simulink model "abs_error"  (R2021b)
settings: Solver=VariableStepAuto  StartTime=0.0  StopTime=10.0  RelTol=1e-3
undefined symbols (not defined in the file): magnitude, Newton, Raphson
libraries: simulink x15
settings Model: PauseTimes=1  Creator=user  LastModifiedBy=cemery

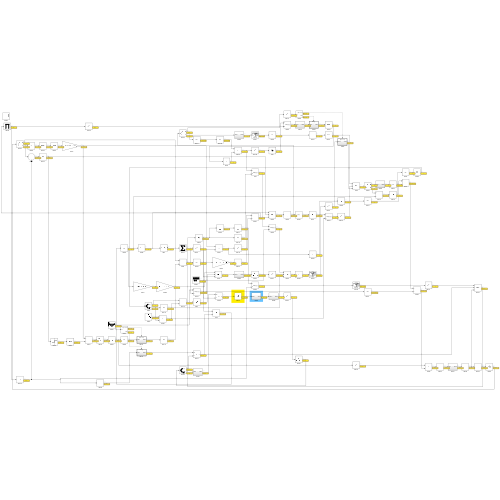
[thumbnail: Simulink's stored preview of the top-level diagram]
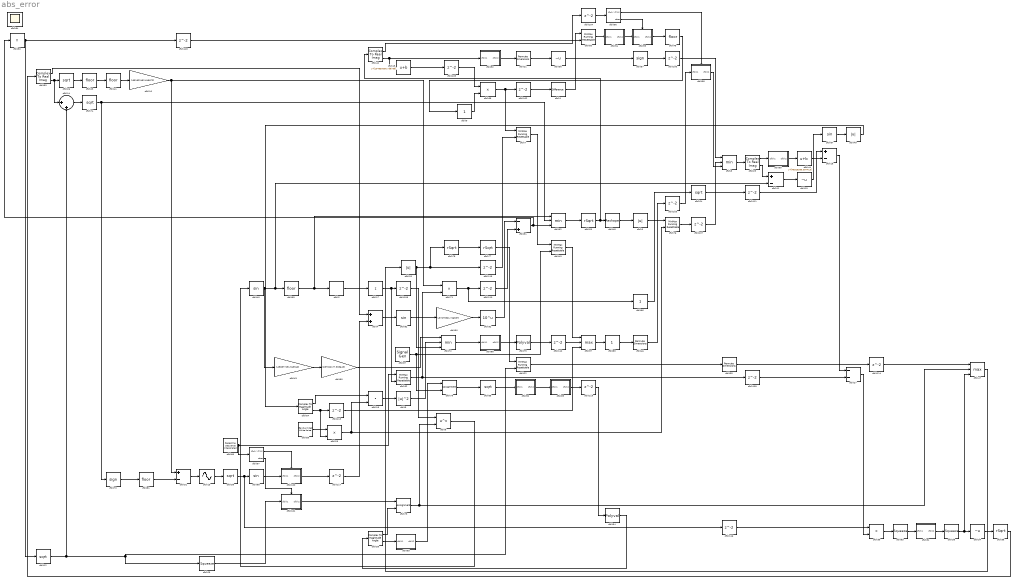
== system abs_error ==
  cfblk1 : simulink/Discrete/Difference  ICPrevInput=0.0  OutMin=[]  OutMax=[]  OutDataTypeStr=Inherit: Inherit via back propagation  OutDataType=fixdt(1, 16)  OutScaling=2^-10  DoSatur=off
  cfblk10 : Gain  Gain=[-531822452.645872]
  cfblk100 : Subsystem  TreatAsAtomicUnit=on
  cfblk101 : Subsystem  TreatAsAtomicUnit=on
  cfblk{102..119} (18 alike) : Delay  SampleTime=1
  cfblk11 : Sum  Inputs=+-
  cfblk{12,24,26,59,65,74} (6 alike) : Sqrt  SaturateOnIntegerOverflow=on
  cfblk13 : Sin  TimeSource=Use external signal  SampleTime=0
  cfblk14 : Sum  Inputs=|++
  cfblk15 : Bias  Bias=[104830006.738759]
  cfblk16 : Sum  Inputs=+-
  cfblk17 : Sum  Inputs=+
  cfblk18 : DotProduct  InputSameDT=on  OutDataTypeStr=Inherit: Inherit via internal rule
  cfblk19 : UnaryMinus
  cfblk2 : DiscreteStateSpace
  cfblk20 : Abs
  cfblk21 : PermuteDimensions
  cfblk{7,22,32,43,60,76} (6 alike) : simulink/Math Operations/MinMax Running Resettable  Function=min  vinit=0.0
  cfblk{23,41,45,69,81} (5 alike) : Rounding
  cfblk25 : Squeeze
  cfblk27 : Sum  Inputs=--
  cfblk28 : Product  Inputs=**
  cfblk29 : ComplexToRealImag
  cfblk3 : Abs
  cfblk30 : Product  Inputs=*
  cfblk31 : Sum  Inputs=-+
  cfblk{33,56,77..78} (4 alike) : Sqrt  Operator=rSqrt  AlgorithmType=Newton-Raphson  SaturateOnIntegerOverflow=on
  cfblk34 : UnaryMinus
  cfblk35 : PermuteDimensions
  cfblk36 : UnaryMinus
  cfblk37 : MinMax  Function=max  Inputs=3
  cfblk38 : Squeeze
  cfblk39 : Product
  cfblk4 : Sum
  cfblk{40,67..68,82} (4 alike) : Trigonometry
  cfblk42 : ComplexToRealImag
  cfblk44 : Bias  Bias=[46526396.097413]
  cfblk46 : PermuteDimensions
  cfblk47 : MinMax  Function=max  Inputs=3
  cfblk48 : Reshape
  cfblk49 : Abs
  cfblk5 : Math  Operator=magnitude^2  SaturateOnIntegerOverflow=on
  cfblk50 : Gain  Gain=[-97079901.726537]
  cfblk51 : Sum  Inputs=+-
  cfblk52 : Math  Operator=10^u  SaturateOnIntegerOverflow=on
  cfblk53 : ComplexToRealImag
  cfblk54 : Polyval  Coefs=[ +2.081618890e-019, -1.441693666e-014, +4.719686976e-010, -8.536869453e-006, +1.621573104e-001, -8.087801117e+001 ]
  cfblk55 : ComplexToMagnitudeAngle
  cfblk57 : Signum
  cfblk58 : Product
  cfblk6 : Math  Operator=pow  SaturateOnIntegerOverflow=on
  cfblk61 : Gain  Gain=[-258877291.943940]
  cfblk62 : MinMax  Inputs=3
  cfblk63 : Squeeze
  cfblk64 : ComplexToMagnitudeAngle
  cfblk66 : simulink/Math Operations/Slider Gain  gain=1  low=0  high=2
  cfblk70 : Signum
  cfblk71 : Product  Inputs=**
  cfblk72 : MinMax  Inputs=3
  cfblk73 : Assignment  DiagnosticForDimensions=Warning  IndexOptions=Index vector (dialog)  Indices=1  OutputSizes=1
  cfblk75 : Polyval  Coefs=[ +2.081618890e-019, -1.441693666e-014, +4.719686976e-010, -8.536869453e-006, +1.621573104e-001, -8.087801117e+001 ]
  cfblk79 : Assignment  DiagnosticForDimensions=Warning  IndexOptions=Index vector (dialog)  Indices=1  OutputSizes=1
  cfblk8 : MinMax  Inputs=3
  cfblk80 : Gain  Gain=[287322177.333645]
  cfblk83 : simulink/Math Operations/Slider Gain  gain=1  low=0  high=2
  cfblk84 : Scope
      settings: Floating=on
  cfblk85 : simulink/Sources/Band-Limited White Noise  Cov=[4231754352.057434]  Ts=0.1  seed=[6656747697.000000]
  cfblk86 : simulink/Sources/Repeating Sequence Interpolated  OutValues=[842062984.296176, 159650378.742997, -714956716.092378, -557171491.799580, 214150598.543998]  TimeValues=[0 0.1 0.5 0.6 1].'  LookUpMeth=Interpolation-Use End Values  tsamp=0.01  OutMin=[]  OutMax=[]  OutDataTypeStr=double  OutputDataTypeScalingMode=double  OutDataType=fixdt(0,8)  OutScaling=2^-10
  cfblk87 : SignalGenerator  WaveForm=square  Amplitude=[478990331.282242]  Units=rad/sec
  cfblk88 : Subsystem
  cfblk89 : Subsystem
  cfblk9 : simulink/Math Operations/Slider Gain  gain=1  low=0  high=2
  cfblk90 : Subsystem
  cfblk91 : Subsystem
  cfblk92 : Subsystem
  cfblk93 : Subsystem
  cfblk94 : Subsystem
  cfblk95 : Subsystem
  cfblk96 : If  IfExpression=u1 >= 0  SampleTime=1
  cfblk97 : If  IfExpression=u1 >= 0  SampleTime=1
  cfblk98 : Subsystem  TreatAsAtomicUnit=on
  cfblk99 : Subsystem  TreatAsAtomicUnit=on
  wires:
  cfblk24/1 -> cfblk111/1
  cfblk114/1 -> cfblk47/1
  cfblk90/1(cfblk2) -> cfblk89/1(cfblk1)
  cfblk117/1 -> cfblk4/2
  cfblk111/1 -> cfblk16/1
  cfblk89/1(cfblk2) -> cfblk119/1
  cfblk35/1 -> cfblk114/1
  cfblk119/1 -> cfblk54/1
  cfblk100/1(cfblk2) -> cfblk117/1
  cfblk115/1 -> cfblk7/2
  cfblk113/1 -> cfblk37/3
  cfblk116/1 -> cfblk39/1
  cfblk118/1 -> cfblk60/2
  cfblk112/1 -> cfblk37/2
  cfblk75/1 -> cfblk112/1
  cfblk1/1 -> cfblk60/1
  cfblk110/1 -> cfblk31/2
  cfblk45/1 -> cfblk9/1
  cfblk109/1 -> cfblk27/2
  cfblk29/2 -> cfblk11/1
  cfblk108/1 -> cfblk6/1
  cfblk107/1 -> cfblk8/2
  cfblk76/1 -> cfblk107/1
  cfblk97/1 -> cfblk100/Action
  cfblk106/1 -> cfblk8/1
  cfblk57/1 -> cfblk106/1
  cfblk105/1 -> cfblk58/1
  cfblk15/1 -> cfblk105/1
  cfblk14/1 -> cfblk74/1
  cfblk64/1 -> cfblk18/1
  cfblk104/1 -> cfblk96/1
  cfblk85/1 -> cfblk28/1
  cfblk98/1(cfblk2) -> cfblk8/3
  cfblk42/1 -> cfblk104/1
  cfblk103/1 -> cfblk98/1(cfblk1)
  cfblk46/1 -> cfblk103/1
  cfblk102/1 -> cfblk1/1
  cfblk61/1 -> cfblk80/1
  cfblk97/2 -> cfblk101/Action
  cfblk81/1 -> cfblk51/2
  cfblk96/2 -> cfblk99/Action
  cfblk19/1 -> cfblk67/1
  cfblk96/1 -> cfblk98/Action
  cfblk95/1(cfblk2) -> cfblk44/1
  cfblk3/1 -> cfblk76/1
  cfblk22/1 -> cfblk35/1
  cfblk88/1(cfblk2) -> cfblk75/1
  cfblk55/2 -> cfblk93/1(cfblk1)
  cfblk50/1 -> cfblk52/1
  cfblk77/1 -> cfblk22/1
  cfblk21/1 -> cfblk36/1
  cfblk29/1 -> cfblk95/1(cfblk1)
  cfblk48/1 -> cfblk3/1
  cfblk27/1 -> cfblk39/2
  cfblk49/1 -> cfblk64/1
  cfblk5/1 -> cfblk72/2
  cfblk7/1 -> cfblk43/1
  cfblk43/1 -> cfblk37/1
  cfblk47/1 -> cfblk20/1
  cfblk25/1 -> cfblk101/1(cfblk1)
  cfblk80/1 -> cfblk72/1
  cfblk6/1 -> cfblk40/1
  cfblk2/1 -> cfblk17/1
  cfblk54/1 -> cfblk55/1
  cfblk91/1(cfblk2) -> cfblk38/1
  cfblk26/1 -> cfblk23/1
  cfblk9/1 -> cfblk58/2
  cfblk44/1 -> cfblk16/2
  cfblk18/1 -> cfblk5/1
  cfblk82/1 -> cfblk50/1
  cfblk60/1 -> cfblk94/1(cfblk1)
  cfblk37/1 -> cfblk83/1
  cfblk53/1 -> cfblk4/1
  cfblk68/1 -> cfblk100/1(cfblk1)
  cfblk55/1 -> cfblk73/2
  cfblk66/1 -> cfblk24/1
  cfblk65/1 -> cfblk90/1(cfblk1)
  cfblk23/1 -> cfblk41/1
  cfblk13/1 -> cfblk59/1
  cfblk101/1(cfblk2) -> cfblk73/1
  cfblk83/1 -> cfblk46/1
  cfblk63/1 -> cfblk91/1(cfblk1)
  cfblk67/1 -> cfblk49/1
  cfblk78/1 -> cfblk77/1
  cfblk39/1 -> cfblk63/1
  cfblk16/1 -> cfblk27/1
  cfblk92/1(cfblk2) -> cfblk21/1
  cfblk11/1 -> cfblk19/1
  cfblk8/1 -> cfblk29/1
  cfblk4/1 -> cfblk82/1
  cfblk36/1 -> cfblk57/1
  cfblk62/1 -> cfblk33/1
  cfblk52/1 -> cfblk31/1
  cfblk56/1 -> cfblk53/1
  cfblk70/1 -> cfblk81/1
  cfblk72/1 -> cfblk88/1(cfblk1)
  cfblk79/1 -> cfblk65/1
  cfblk41/1 -> cfblk10/1
  cfblk94/1(cfblk2) -> cfblk99/1(cfblk1)
  cfblk51/1 -> cfblk13/1
  cfblk34/1 -> cfblk56/1
  cfblk99/1(cfblk2) -> cfblk45/1
  cfblk93/1(cfblk2) -> cfblk79/1
  cfblk42/2 -> cfblk15/1, cfblk92/1(cfblk1)
  cfblk10/1 -> cfblk51/1, cfblk71/1
  cfblk86/1 -> cfblk97/1, cfblk32/1
  cfblk64/2 -> cfblk28/2, cfblk113/1
  cfblk31/1 -> cfblk30/1, cfblk62/3
  cfblk20/1 -> cfblk115/1, cfblk78/1, cfblk72/3
  cfblk28/1 -> cfblk76/2, cfblk18/2
  cfblk38/1 -> cfblk34/1, cfblk47/3
  cfblk53/2 -> cfblk26/1, cfblk14/1
  cfblk58/1 -> cfblk7/1, cfblk102/1
  cfblk73/1 -> cfblk6/2, cfblk47/2
  cfblk32/1 -> cfblk71/2, cfblk109/1
  cfblk17/1 -> cfblk32/2, cfblk108/1
  cfblk69/1 -> cfblk62/1, cfblk2/1
  cfblk33/1 -> cfblk42/1, cfblk48/1
  cfblk71/1 -> cfblk66/1, cfblk110/1
  cfblk59/1 -> cfblk68/1, cfblk116/1
  cfblk87/1 -> cfblk79/2, cfblk43/2
  cfblk40/1 -> cfblk69/1, cfblk11/2, cfblk61/1
  cfblk12/1 -> cfblk25/1, cfblk22/2, cfblk14/2
  cfblk30/1 -> cfblk12/1, cfblk118/1
  cfblk74/1 -> cfblk70/1, cfblk62/2

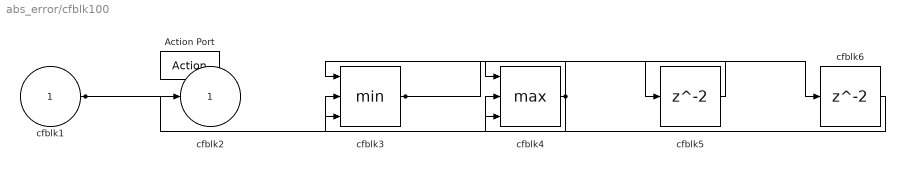
== system abs_error/cfblk100 ==
  cfblk1 : Inport
  Action Port : ActionPort  ActionPortLabel=if(u1 >= 0)
  cfblk3 : MinMax  Inputs=3
  cfblk4 : MinMax  Function=max  Inputs=3
  cfblk5 : Delay
  cfblk6 : Delay
  cfblk2 : Outport
  wires:
  cfblk1/1 -> cfblk2/1, cfblk4/2
  cfblk4/1 -> cfblk3/1, cfblk3/2, cfblk3/3
  cfblk3/1 -> cfblk5/1, cfblk6/1
  cfblk5/1 -> cfblk4/1
  cfblk6/1 -> cfblk4/3

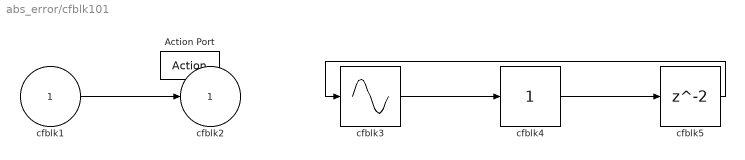
== system abs_error/cfblk101 ==
  cfblk1 : Inport
  Action Port : ActionPort  ActionPortLabel=else
  cfblk3 : Sin  TimeSource=Use external signal  SampleTime=0
  cfblk4 : simulink/Math Operations/Slider Gain  gain=1  low=0  high=2
  cfblk5 : Delay
  cfblk2 : Outport
  wires:
  cfblk3/1 -> cfblk4/1
  cfblk1/1 -> cfblk2/1
  cfblk4/1 -> cfblk5/1
  cfblk5/1 -> cfblk3/1

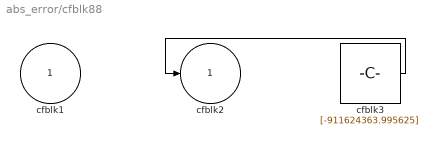
== system abs_error/cfblk88 ==
  cfblk1 : Inport
  cfblk3 : Constant  Value=[-911624363.995625]  SampleTime=1
  cfblk2 : Outport
  wires:
  cfblk3/1 -> cfblk2/1

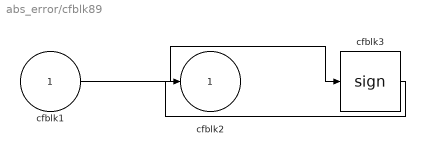
== system abs_error/cfblk89 ==
  cfblk1 : Inport
  cfblk3 : Signum
  cfblk2 : Outport
  wires:
  cfblk1/1 -> cfblk3/1
  cfblk3/1 -> cfblk2/1

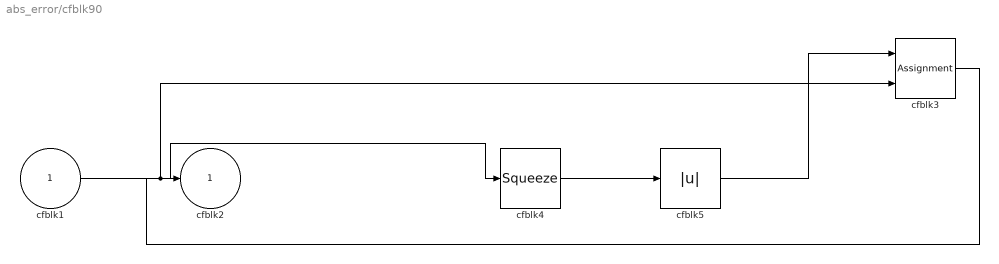
== system abs_error/cfblk90 ==
  cfblk1 : Inport
  cfblk3 : Assignment  DiagnosticForDimensions=Warning  IndexOptions=Index vector (dialog)  Indices=1  OutputSizes=1
  cfblk4 : Squeeze
  cfblk5 : Abs
  cfblk2 : Outport
  wires:
  cfblk1/1 -> cfblk4/1, cfblk3/2
  cfblk4/1 -> cfblk5/1
  cfblk5/1 -> cfblk3/1
  cfblk3/1 -> cfblk2/1

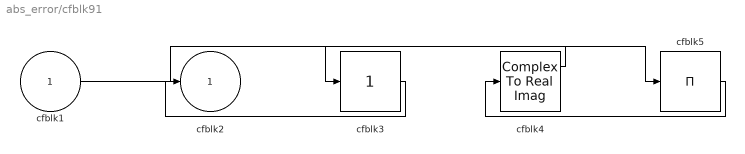
== system abs_error/cfblk91 ==
  cfblk1 : Inport
  cfblk3 : simulink/Math Operations/Slider Gain  gain=1  low=0  high=2
  cfblk4 : ComplexToRealImag
  cfblk5 : Product  Inputs=*
  cfblk2 : Outport
  wires:
  cfblk1/1 -> cfblk5/1
  cfblk5/1 -> cfblk4/1
  cfblk4/1 -> cfblk3/1
  cfblk3/1 -> cfblk2/1

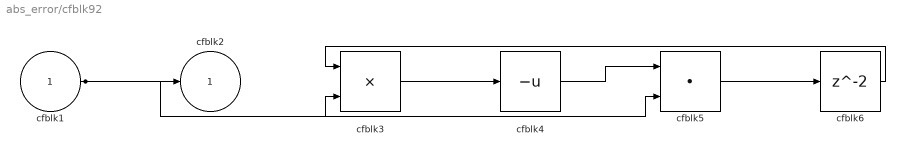
== system abs_error/cfblk92 ==
  cfblk1 : Inport
  cfblk3 : Product
  cfblk4 : UnaryMinus
  cfblk5 : DotProduct  InputSameDT=on  OutDataTypeStr=Inherit: Inherit via internal rule
  cfblk6 : Delay  SampleTime=1
  cfblk2 : Outport
  wires:
  cfblk1/1 -> cfblk2/1, cfblk3/2, cfblk5/2
  cfblk3/1 -> cfblk4/1
  cfblk4/1 -> cfblk5/1
  cfblk5/1 -> cfblk6/1
  cfblk6/1 -> cfblk3/1

== system abs_error/cfblk93 ==
  cfblk1 : Inport
  cfblk3 : Polyval  Coefs=[ +2.081618890e-019, -1.441693666e-014, +4.719686976e-010, -8.536869453e-006, +1.621573104e-001, -8.087801117e+001 ]
  cfblk2 : Outport
  wires:
  cfblk3/1 -> cfblk2/1
  cfblk1/1 -> cfblk3/1

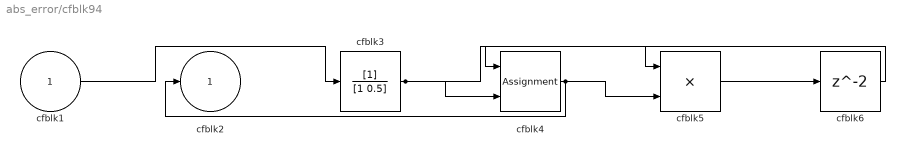
== system abs_error/cfblk94 ==
  cfblk1 : Inport
  cfblk3 : DiscreteFilter  SampleTime=1
  cfblk4 : Assignment  DiagnosticForDimensions=Warning  IndexOptions=Index vector (dialog)  Indices=1  OutputSizes=1
  cfblk5 : Product
  cfblk6 : Delay  SampleTime=1
  cfblk2 : Outport
  wires:
  cfblk3/1 -> cfblk4/2, cfblk5/1
  cfblk4/1 -> cfblk2/1, cfblk5/2
  cfblk1/1 -> cfblk3/1
  cfblk5/1 -> cfblk6/1
  cfblk6/1 -> cfblk4/1

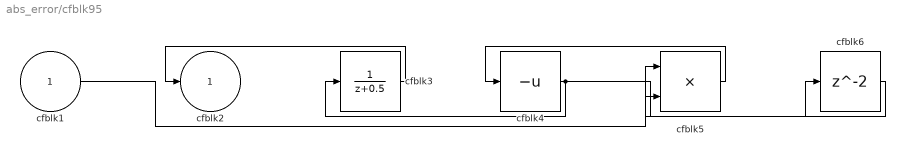
== system abs_error/cfblk95 ==
  cfblk1 : Inport
  cfblk3 : DiscreteTransferFcn  SampleTime=1
  cfblk4 : UnaryMinus
  cfblk5 : Product
  cfblk6 : Delay  SampleTime=1
  cfblk2 : Outport
  wires:
  cfblk5/1 -> cfblk4/1
  cfblk4/1 -> cfblk3/1, cfblk6/1
  cfblk3/1 -> cfblk2/1
  cfblk1/1 -> cfblk5/1
  cfblk6/1 -> cfblk5/2

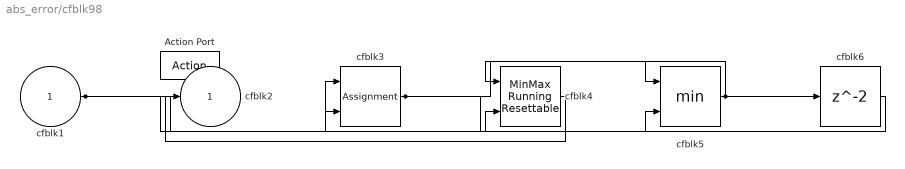
== system abs_error/cfblk98 ==
  cfblk1 : Inport
  Action Port : ActionPort  ActionPortLabel=if(u1 >= 0)
  cfblk3 : Assignment  DiagnosticForDimensions=Warning  IndexOptions=Index vector (dialog)  Indices=1  OutputSizes=1
  cfblk4 : simulink/Math Operations/MinMax Running Resettable  Function=min  vinit=0.0
  cfblk5 : MinMax  Inputs=2
  cfblk6 : Delay
  cfblk2 : Outport
  wires:
  cfblk3/1 -> cfblk5/1, cfblk5/2
  cfblk1/1 -> cfblk3/1, cfblk4/2
  cfblk4/1 -> cfblk2/1
  cfblk5/1 -> cfblk4/1, cfblk6/1
  cfblk6/1 -> cfblk3/2

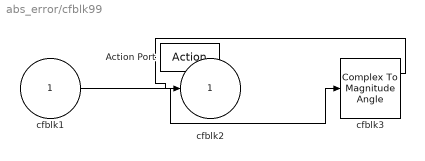
== system abs_error/cfblk99 ==
  cfblk1 : Inport
  Action Port : ActionPort  ActionPortLabel=else
  cfblk3 : ComplexToMagnitudeAngle
  cfblk2 : Outport
  wires:
  cfblk1/1 -> cfblk3/1
  cfblk3/1 -> cfblk2/1
